simulink model "mav_project"  (R2024b)
settings: Solver=ode4  StartTime=0.0  StopTime=10000  RelTol=1e-3  EnableMultiTasking=on
model workspace (MAT data in the model file):
  P.gravity = 9.8
  P.mass = 1.56
  P.Jx = 0.1147
  P.Jy = 0.0576
  P.Jz = 0.1712
  P.Jxz = 0.0015
  P.M = 50
  P.epsilon = 0.1592
  P.alpha0 = 0.4712
  P.rho = 1.2682
  P.c = 0.3302
  P.b = 1.4224
  P.S_wing = 0.2589
  P.S_prop = 0.0314
  P.k_motor = 20
  P.C_L_0 = 0.28
  P.C_L_alpha = 3.45
  P.C_L_q = 0
  P.C_L_delta_e = -0.36
  P.C_D_0 = 0.03
  P.C_D_q = 0
  P.C_D_delta_e = 0
  P.C_M_0 = 0
  P.C_M_alpha = -0.38
  P.C_M_q = -3.6
  P.C_M_delta_e = -0.5
  P.C_Y_0 = 0
  P.C_Y_beta = -0.98
  P.C_Y_p = -0.26
  P.C_Y_r = 0
  P.C_Y_delta_a = 0
  P.C_Y_delta_r = -0.17
  P.C_ell_0 = 0
  P.C_ell_beta = -0.12
  P.C_ell_p = -0.26
  P.C_ell_r = 0.14
  P.C_ell_delta_a = 0.08
  P.C_ell_delta_r = 0.105
  P.C_n_0 = 0
  P.C_n_beta = 0.25
  P.C_n_p = 0.022
  P.C_n_r = -0.35
  P.C_n_delta_a = 0.06
  P.C_n_delta_r = -0.032
  P.C_prop = 1
  P.wind_n = 0
  P.wind_e = 0
  P.wind_d = 0
  P.L_wx = 1250
  P.L_wy = 1750
  P.L_wz = 1750
  P.sigma_wx = 1
  P.sigma_wy = 1
  P.sigma_wz = 1
  P.Va0 = 10
  P.Ts = 0.01
  P.Va = 13
  P.pn0 = 0
  P.pe0 = 0
  P.pd0 = 0
  P.u0 = 12.9669102518
  P.v0 = 3.28039918827e-26
  P.w0 = 0.926951196428
  P.phi0 = 1.93188396575e-23
  P.theta0 = 0.0713644980387
  P.psi0 = 4.37095971631e-18
  P.p0 = -4.12839964336e-24
  P.q0 = -1.29183976294e-24
  P.r0 = 9.37982436998e-24
  P.u_trim = [-0.0542370185094; 4.00408429765e-25; -1.10117211384e-23; 0.825366374251]
  P.x_trim = [5.38381030697e-18; -2.86631315328e-18; 3.31364444525e-19; 12.9669102518; 3.28039918827e-26; 0.926951196428; 1.93188396575e-23; 0.0713644980387; 4.37095971631e-18; -4.12839964336e-24; -1.29183976294e-24; 9.37982436998e-24]
  P.tau = 5
  P.altitude_take_off_zone = 10
  P.altitude_hold_zone = 10
  P.roll_kp = 2.56718517289
  P.roll_kd = 0.253887920845
  P.roll_ki = 0.1
  P.heading_kp = 1.58199403044
  P.heading_ki = 0.943612282481
  P.heading_kd = 0
  P.beta_kp = 0.116355283466
  P.beta_ki = 0
  P.beta_kd = 0
  P.pitch_kp = -1.36164063875
  P.pitch_kd = -0.139518937604
  P.pitch_ki = 0
  P.K_theta_DC = 0.641786650331
  P.altitude_kp = 0.0733804862104
  P.altitude_ki = 0.0224696538774
  P.altitude_kd = 0
  P.airspeed_pitch_kp = -0.208266228183
  P.airspeed_pitch_ki = -0.268260153434
  P.airspeed_pitch_kd = 0
  P.airspeed_throttle_kp = 12.4207118815
  P.airspeed_throttle_ki = 2.96647332332
  P.airspeed_throttle_kd = 0
  P.sideslip_kp = 0.1
  P.sideslip_kd = -0.5
  P.sideslip_ki = 0
values from neighbouring files (symbols this model uses):
  P = varargin{5}    [my_mav_dynamics.m]
undefined symbols (not defined in the file or in its folder): autopilot, drawAircraft, ekf_nav, forces_moments, gps_sensor, Guidance, imu_sensor, LQR_Controller, plotmavstatevariables, Receive, Send
libraries: simulink x6, aerolibanim x2, aerolibfltsims x2, slrealtimeiplib x1, vrlib x1
settings Model: SimulationMode=accelerator  Creator=beard  LastModifiedBy=solot
settings SolverCC: AutoInsertRateTranBlk=on
settings DataIOCC: LimitDataPoints=on  SaveFormat=Array  SignalLoggingSaveFormat=ModelDataLogs  ReturnWorkspaceOutputs=off
settings OptimizationCC: ExpressionDepthLimit=2147483647  InitFltsAndDblsToZero=on  LifeSpan=inf
settings DebuggingCC: SolverPrmCheckMsg=warning  FcnCallInpInsideContextMsg=warning  UnconnectedInputMsg=warning  UnconnectedOutputMsg=warning  UnconnectedLineMsg=warning  StateNameClashWarn=warning  SFUnexpectedBacktrackingDiag=warning  SFNoUnconditionalDefaultTransitionDiag=warning  SFExecutionAtInitializationDiag=none  ArithmeticOperatorsInVariantConditions=warning
settings HardwareCC: ProdBitPerPointer=32  ProdBitPerSizeT=32  ProdBitPerPtrDiffT=32  ProdLargestAtomicFloat=None  ProdIntDivRoundTo=Undefined  ProdEndianess=Unspecified  ProdWordSize=32  ProdHWDeviceType=32-bit Generic
settings ModelReferenceCC: EnableRefExpFcnMdlSchedulingChecks=on  PropagateSignalLabelsOutOfModel=off
settings SFSimCC: SimUseLocalCustomCode=off  CustomCodeUndefinedFunction=UseInterfaceOnly
settings RTWCC: RTWUseLocalCustomCode=off  GPUComputeCapability=3.5  DLArmComputeVersion=19.05
settings CodeAppCC: StateflowObjectComments=on
settings GRTTargetCC: TargetLangStandard=C89/C90 (ANSI)  CombineOutputUpdateFcns=off  GRTInterface=on
settings ConfigComp: CovMetricSettings=dw  CovSaveCumulativeToWorkspaceVar=on  CovSaveSingleToWorkspaceVar=on  CovExternalEMLEnable=off

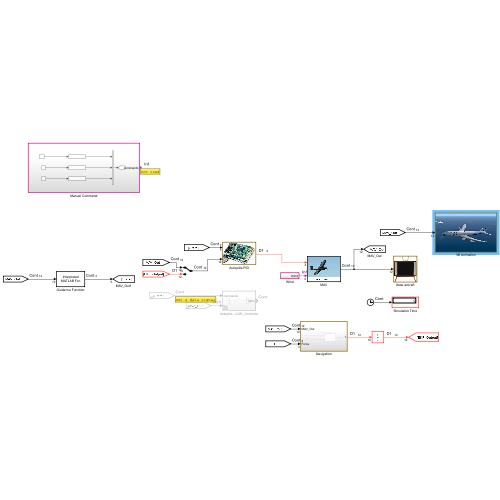
[thumbnail: Simulink's stored preview of the top-level diagram]
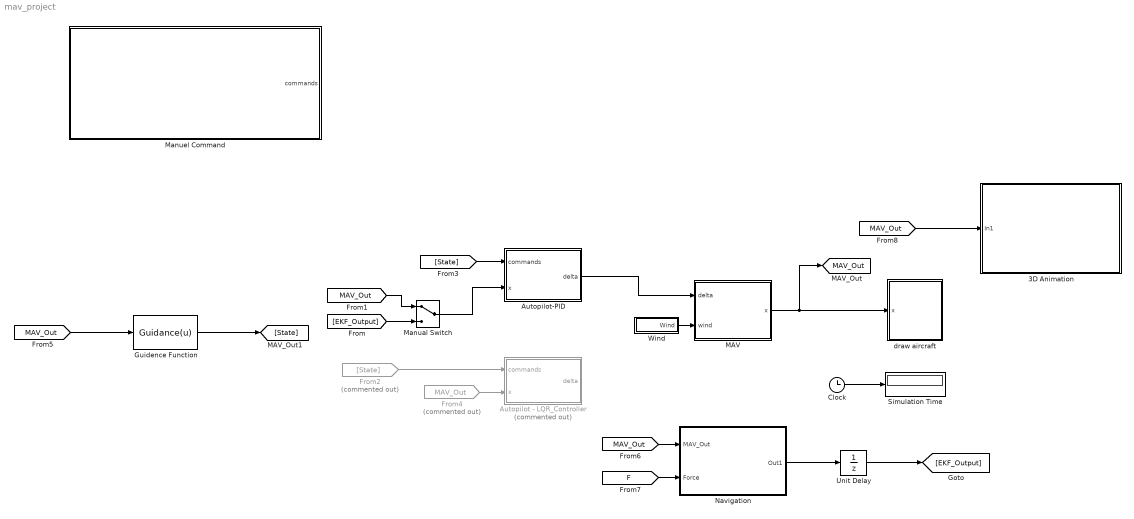
== system mav_project ==
  3D Animation : Subsystem
      mask Display: image(imread('flight.jpg'))
  Autopilot - LQR_Controller : Subsystem  Commented=on
  Autopilot-PID : Subsystem
      mask Display: image('kestrel.jpg')
  Clock : Clock
  From2 : From  Commented=on  GotoTag=State
  From4 : From  Commented=on  GotoTag=MAV_Out  TagVisibility=global
  Guidence Function : MATLABFcn  MATLABFcn=Guidance(u)  OutputDimensions=3
  MAV : Subsystem
      mask Display: image('batcam.png')
  Manual Switch : ManualSwitch
  "Manuel Command " : Subsystem
  Navigation : Subsystem
  Simulation Time : Display
  Unit Delay : UnitDelay  SampleTime=0.01  HasFrameUpgradeWarning=on
  Wind : Subsystem
  draw aircraft : Subsystem
      mask init:
      | % parameters for drawing aircraft
      |   % scale size
      |   size = 20;
      |   fuse_l1    = 7;
      |   fuse_l2    = 4;
      |   fuse_l3    = 15;
      |   fuse_w     = 2;
      |   wing_l     = 6;
      |   wing_w     = 20;
      |   tail_l     = 3;
      |   tail_h     = 3;
      |   tailwing_w = 10;
      |   tailwing_l = 3;
      |   % colors
      |   red     = [1, 0, 0];
      |   green   = [0, 1, 0];
      |   blue    = [0, 0, 1];
      |   yellow  = [1,1,0];
      |   magenta = [0, 1, 1];
      |   
      | 
      | % define vertices and faces for aircraft
      |   V = [...
      |     fuse_l1,             0,             0;...        % point 1
      |     fuse_l2,            -fuse_w/2,     -fuse_w/2;... % point 2     
      |     fuse_l2,             fuse_w/2,     -fuse_w/2;... % point 3     
      |     fuse_l2,             fuse_w/2,      fuse_w/2;... % point 4
      |     fuse_l2,            -fuse_w/2,      fuse_w/2;... % point 5
      |    -fuse_l3,             0,             0;...        % point 6
      |     0,                   wing_w/2,      0;...        % point 7
      |    -wing_l,              wing_w/2,      0;...        % point 8
      |    -wing_l,             -wing_w/2,      0;...        % point 9
      |     0,                  -wing_w/2,      0;...        % point 10
      |    -fuse_l3+tailwing_l,  tailwing_w/2,  0;...        % point 11
      |    -fuse_l3,             tailwing_w/2,  0;...        % point 12
      |    -fuse_l3,            -tailwing_w/2,  0;...        % point 13
      |    -fuse_l3+tailwing_l, -tailwing_w/2,  0;...        % point 14
      |    -fuse_l3+tailwing_l,  0,             0;...        % point 15
      |    -fuse_l3+tailwing_l,  0,             -tail_h;...  % point 16
      |    -fuse_l3,             0,             -tail_h;...  % point 17
      |   ];
      |   
      |   F = [...
      |         1,  2,  3,  1;... % nose-top
      |         1,  3,  4,  1;... % nose-left
      |         1,  4,  5,  1;... % nose-bottom
      |         1,  5,  2,  1;... % nose-right
      |         2,  3,  6,  2;... % fuselage-top
      |         3,  6,  4,  3;... % fuselage-left
      |         4,  6,  5,  4;... % fuselage-bottom
      |         2,  5,  6,  2;... % fuselage-right
      |         7,  8,  9, 10;... % wing
      |        11, 12, 13, 14;... % tailwing
      |         6, 15, 17, 17;... % tail
      |         
      |   ];  
      |   
      |   colors = [...
      |         yellow;... % nose-top
      |         yellow;... % nose-left
      |         yellow;... % nose-bottom
      |         yellow;... % nose-right
      |         blue;... % fuselage-top
      |         blue;... % fuselage-left
      |         red;... % fuselage-bottom
      |         blue;... % fuselage-right
      |         green;... % wing
      |         green;... % tailwing
      |         blue;... % tail
      |     ];
      | 
      |   V = size*V;   % rescale vertices
      mask Display: image('tv.jpg')
  tag scope: MAV_Out=global
  wires:
  Clock/1 -> Simulation Time/1
  Wind/1(Wind) -> MAV/2(wind)
  MAV/1(x) -> [MAV_Out], draw aircraft/1(x)
  [MAV_Out] -> Guidence Function/1
  From4/1 -> Autopilot - LQR_Controller/2(x)
  Guidence Function/1 -> [State]
  [MAV_Out] -> Navigation/1(MAV_Out)
  [F] -> Navigation/2(Force)
  Navigation/1(Out1) -> Unit Delay/1
  Unit Delay/1 -> [EKF_Output]
  [State] -> Autopilot-PID/1(commands)
  Manual Switch/1 -> Autopilot-PID/2(x)
  [EKF_Output] -> Manual Switch/2
  [MAV_Out] -> Manual Switch/1
  From2/1 -> Autopilot - LQR_Controller/1(commands)
  Autopilot-PID/1(delta) -> MAV/1(delta)
  [MAV_Out] -> 3D Animation/1(In1)

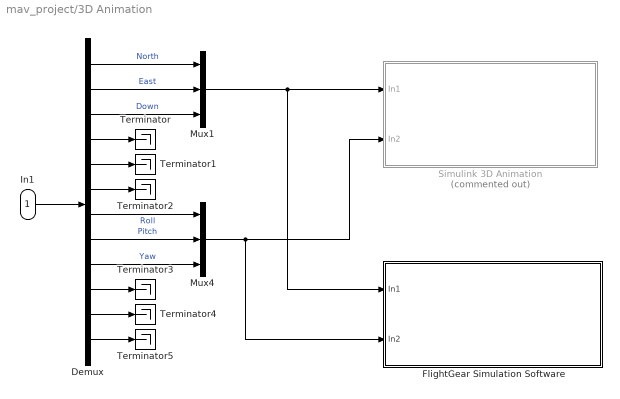
== system mav_project/3D Animation ==
  In1 : Inport
  Demux : Demux  Outputs=12
  FlightGear Simulation Software : Subsystem
      mask Display: image(imread('flightgear.jpg'))
  Mux1 : Mux  Inputs=3
  Mux4 : Mux  Inputs=3
  Simulink 3D Animation : Subsystem  Commented=on
      mask Display: image(imread('3danimation.JPG'))
  Terminator{,1..5} (6 alike) : Terminator
  wires:
  In1/1 -> Demux/1
  Demux/4 -> Terminator/1
  Demux/5 -> Terminator1/1
  Demux/6 -> Terminator2/1
  Demux/10 -> Terminator3/1
  Demux/11 -> Terminator4/1
  Demux/12 -> Terminator5/1
  Demux/1 -> Mux1/1  "North"
  Demux/2 -> Mux1/2  "East"
  Demux/3 -> Mux1/3  "Down"
  Mux1/1 -> FlightGear Simulation Software/1(In1), Simulink 3D Animation/1(In1)
  Demux/7 -> Mux4/1  "Roll"
  Demux/8 -> Mux4/2  "Pitch"
  Demux/9 -> Mux4/3  "Yaw"
  Mux4/1 -> FlightGear Simulation Software/2(In2), Simulink 3D Animation/2(In2)

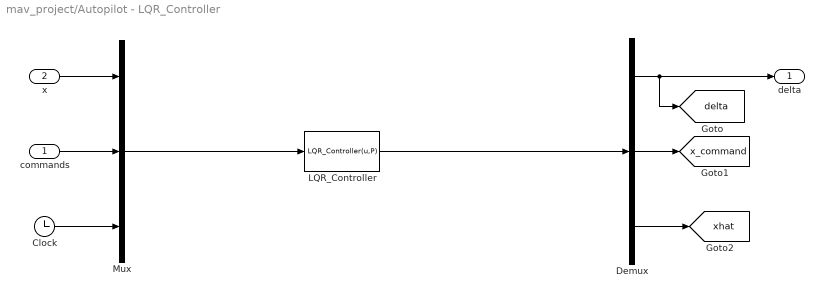
== system mav_project/Autopilot - LQR_Controller ==
  commands : Inport
  x : Inport  Port=2
  Clock : Clock
  Demux : Demux  Outputs=[4;12;12]
  LQR_Controller : MATLABFcn  MATLABFcn=LQR_Controller(u,P)  OutputDimensions=4+12+12
  Mux : Mux  Inputs=3
  delta : Outport
  tag scope: delta=global, x_command=global, xhat=global
  wires:
  Mux/1 -> LQR_Controller/1
  Demux/1 -> delta/1, [delta]
  Demux/3 -> [xhat]
  Demux/2 -> [x_command]
  Clock/1 -> Mux/3
  LQR_Controller/1 -> Demux/1
  commands/1 -> Mux/2
  x/1 -> Mux/1

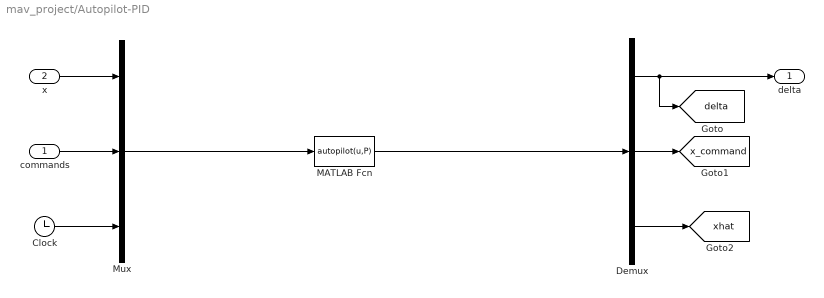
== system mav_project/Autopilot-PID ==
  commands : Inport
  x : Inport  Port=2
  Clock : Clock
  Demux : Demux  Outputs=[4;12;12]
  MATLAB Fcn : MATLABFcn  MATLABFcn=autopilot(u,P)  OutputDimensions=4+12+12  SampleTime=P.Ts
  Mux : Mux  Inputs=3
  delta : Outport
  tag scope: delta=global, x_command=global, xhat=global
  wires:
  Mux/1 -> MATLAB Fcn/1
  Clock/1 -> Mux/3
  MATLAB Fcn/1 -> Demux/1
  Demux/1 -> delta/1, [delta]
  Demux/2 -> [x_command]
  Demux/3 -> [xhat]
  x/1 -> Mux/1
  commands/1 -> Mux/2

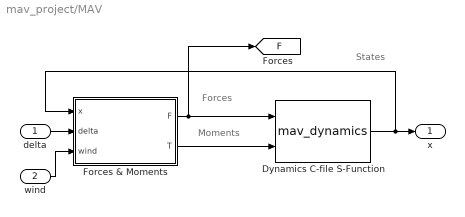
== system mav_project/MAV ==
  note: Forces
  note: Moments
  note: States
  delta : Inport
  wind : Inport  Port=2
  Dynamics C-file S-Function : S-Function  FunctionName=mav_dynamics  Parameters=mass,Jx,Jy,Jz,Jxz,pn0,pe0,pd0,u0,v0,w0,phi0,theta0,psi0,p0,q0,r0  SFunctionDeploymentMode=off  EnableBusSupport=off  mask{mass=P.mass, Jx=P.Jx, Jy=P.Jy, Jz=P.Jz, Jxz=P.Jxz, pn0=P.pn0, pe0=P.pe0, pd0=P.pd0, u0=P.u0, v0=P.v0, w0=P.w0, phi0=P.phi0, theta0=P.theta0, psi0=P.psi0, p0=P.p0, q0=P.q0, r0=P.r0}
      mask prompts: pn0 "Initial North position"; pe0 "Initial East position"; pd0 "Initial Down position"; u0 "Initial velocy u0"; v0 "Initial velocity v0"; w0 "Initial velocity w0"; phi0 "Initial roll angle"; theta0 "Initial pitch angle"; psi0 "Initial yaw angle"; p0 "Initial roll rate"; q0 "Initial pitch rate"; r0 "Initial yaw rate"
  Forces & Moments : Subsystem
  x : Outport
  tag scope: F=global
  wires:
  Dynamics C-file S-Function/1 -> Forces & Moments/1(x), x/1
  Forces & Moments/1(F) -> [F], Dynamics C-file S-Function/1
  Forces & Moments/2(T) -> Dynamics C-file S-Function/2
  delta/1 -> Forces & Moments/2(delta)
  wind/1 -> Forces & Moments/3(wind)

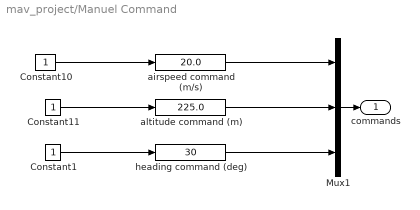
== system mav_project/Manuel Command  ==
  Constant1 : Constant
  Constant10 : Constant
  Constant11 : Constant
  Mux1 : Mux  Inputs=3
  airspeed command (m/s) : simulink/Math Operations/Slider Gain  gain=20.0  low=0  high=20
  altitude command (m) : simulink/Math Operations/Slider Gain  gain=225.0  low=0  high=500
  heading command (deg) : simulink/Math Operations/Slider Gain  gain=30  low=-360  high=360
  commands : Outport
  wires:
  Constant11/1 -> altitude command (m)/1
  heading command (deg)/1 -> Mux1/3
  Constant10/1 -> airspeed command (m/s)/1
  Mux1/1 -> commands/1
  altitude command (m)/1 -> Mux1/2
  airspeed command (m/s)/1 -> Mux1/1
  Constant1/1 -> heading command (deg)/1

== system mav_project/Navigation ==
  MAV_Out : Inport
  Force : Inport  Port=2
  Pulse Generator : DiscretePulseGenerator  PulseType=Time based  Period=1  PulseWidth=50
  Triggered Subsystem : Subsystem  TreatAsAtomicUnit=on
  Out1 : Outport
  wires:
  Pulse Generator/1 -> Triggered Subsystem/Trigger
  MAV_Out/1 -> Triggered Subsystem/1(MAV_Out)
  Force/1 -> Triggered Subsystem/2(Force)
  Triggered Subsystem/1(Out1) -> Out1/1

== system mav_project/Wind ==
  Constant1 : Constant  Value=[0; 0; 0]
  Constant2 : Constant  Value=[P.wind_n; P.wind_e; P.wind_d]
  Mux1 : Mux  Inputs=2
  Wind Gusts : Subsystem  Commented=on
  Wind : Outport
  wires:
  Constant2/1 -> Mux1/1
  Mux1/1 -> Wind/1
  Constant1/1 -> Mux1/2

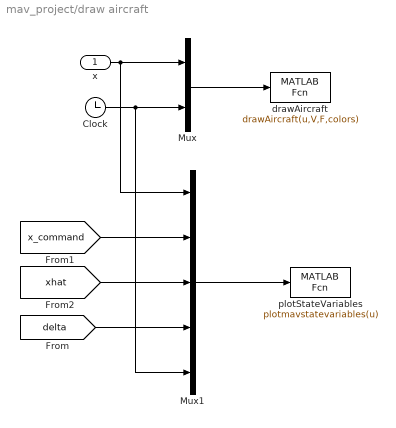
== system mav_project/draw aircraft ==
  x : Inport
  Clock : Clock
  Mux : Mux  Inputs=2
  Mux1 : Mux  Inputs=5
  drawAircraft : MATLABFcn  MATLABFcn=drawAircraft(u,V,F,colors)  OutputDimensions=0  SampleTime=0.1
  plotStateVariables : MATLABFcn  MATLABFcn=plotmavstatevariables(u)  OutputDimensions=0  SampleTime=0.1
  wires:
  Mux/1 -> drawAircraft/1
  x/1 -> Mux/1, Mux1/1
  Clock/1 -> Mux/2, Mux1/5
  Mux1/1 -> plotStateVariables/1
  [xhat] -> Mux1/3
  [x_command] -> Mux1/2
  [delta] -> Mux1/4

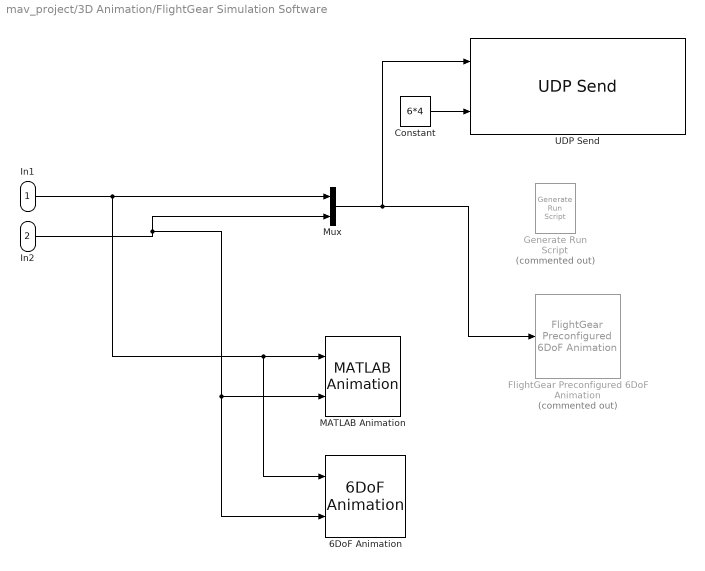
== system mav_project/3D Animation/FlightGear Simulation Software ==
  In1 : Inport
  In2 : Inport  Port=2
  6DoF Animation : aerolibanim/6DoF Animation  u1=[0 4000 -2000 2000 -5000 -3000]  u2=0.1  u3=1.0  u4=[4000 0 -5000]  u5=Fixed position  u6=[2000 500 -3150]  u7=10  u8=on
  Constant : Constant  Value=6*4
  FlightGear Preconfigured 6DoF Animation : aerolibfltsims/FlightGear Preconfigured 6DoF Animation  Commented=on  xFlightGearVersion=v2016.1  DestinationIpAddress=127.0.0.1  DestinationPort=5502  SampleTime=1/100  packetVersion=24
  Generate Run Script : aerolibfltsims/Generate Run Script  Commented=on  Architecture=Default  dataFlow=Send-Receive  GeometryModelName=c172p  AirportId=KSFO  RunwayId=10L  InitialAltitude=7224  InitialHeading=113  OffsetDistance=4.72  OffsetAzimuth=0  InstallScenery=off  DisableShaders=off  OriginAddress=127.0.0.1  DestinationPort=5502  OriginPort=5505  LocalAddress=127.0.0.1  OutputFileName=runfg.bat  FlightGearBaseDirectory=C:\Program Files\FlightGear 2024.1
  MATLAB Animation : aerolibanim/MATLAB Animation  Tag=Matlab Animation 6 DOF  Vehicles=1  Geometries='astredwedge.mat'  BoundingBoxCoordinates=[-50,50,-50,50,-50,50]  CameraOffset=[-150,-50,0]  CameraViewAngle=3  SampleTime=0.2  FigurePosition=[5.482000e+02,1.778000e+02,3.816000e+02,3.352000e+02]
  Mux : Mux  Inputs=2
  UDP Send : slrealtimeiplib/UDP Send  useHostTargetConn=off  toAddress='127.0.0.1'  toPort=5502  sampleTime=0.01  enableMessage=off
  wires:
  In2/1 -> 6DoF Animation/2, MATLAB Animation/2, Mux/2
  In1/1 -> Mux/1, 6DoF Animation/1, MATLAB Animation/1
  Mux/1 -> UDP Send/1, FlightGear Preconfigured 6DoF Animation/1
  Constant/1 -> UDP Send/2

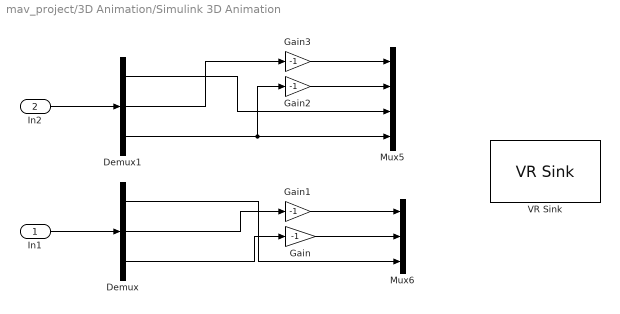
== system mav_project/3D Animation/Simulink 3D Animation ==
  In1 : Inport
  In2 : Inport  Port=2
  Demux : Demux  Outputs=3
  Demux1 : Demux  Outputs=3
  Gain{,1..3} (4 alike) : Gain  Gain=-1
  Mux5 : Mux
  Mux6 : Mux  Inputs=3
  VR Sink : vrlib/VR Sink  InstantiateOnLoad=on  SampleTime=0.05  ViewEnable=on  RemoteChange=off  RemoteView=off  WorldFileName=b748.wrl  WorldDescription=B747 Flying over the San Francisco Area  AutoView=on  VideoDimensions=[]  AllowVariableSize=off
  wires:
  Gain3/1 -> Mux5/1
  Gain1/1 -> Mux6/1
  Gain2/1 -> Mux5/2
  Gain/1 -> Mux6/2
  Demux/3 -> Gain/1
  Demux1/3 -> Gain2/1, Mux5/4
  Demux1/2 -> Gain3/1
  Demux1/1 -> Mux5/3
  Demux/1 -> Mux6/3
  Demux/2 -> Gain1/1
  In1/1 -> Demux/1
  In2/1 -> Demux1/1

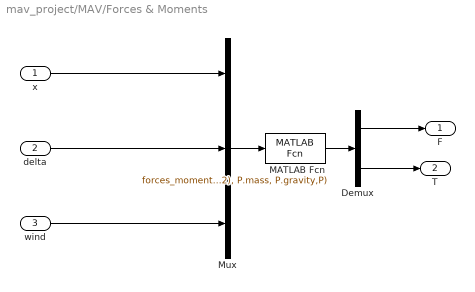
== system mav_project/MAV/Forces & Moments ==
  x : Inport
  delta : Inport  Port=2
  wind : Inport  Port=3
  Demux : Demux  Outputs=2
  MATLAB Fcn : MATLABFcn  MATLABFcn=forces_moments(u(1:12),u(13:16),u(17:22), P.mass, P.gravity,P)  OutputDimensions=6
  Mux : Mux  Inputs=3
  F : Outport
  T : Outport  Port=2
  wires:
  x/1 -> Mux/1
  delta/1 -> Mux/2
  wind/1 -> Mux/3
  MATLAB Fcn/1 -> Demux/1
  Demux/1 -> F/1
  Demux/2 -> T/1
  Mux/1 -> MATLAB Fcn/1

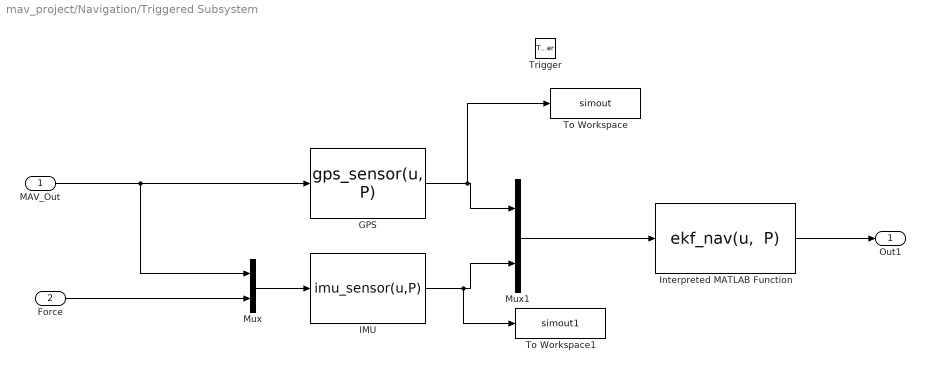
== system mav_project/Navigation/Triggered Subsystem ==
  MAV_Out : Inport
  Force : Inport  Port=2
  Trigger : TriggerPort  VariantControl=(inherit)
  GPS : MATLABFcn  MATLABFcn=gps_sensor(u, P)  OutputDimensions=5
  IMU : MATLABFcn  MATLABFcn=imu_sensor(u,P)  OutputDimensions=6
  Interpreted MATLAB Function : MATLABFcn  MATLABFcn="ekf_nav(u,  P)"  OutputDimensions=12
  Mux : Mux  Inputs=2
  Mux1 : Mux  Inputs=2
  To Workspace : ToWorkspace  VariableName=simout  SaveFormat=Structure  SampleTime=-1
  To Workspace1 : ToWorkspace  VariableName=simout1  SaveFormat=Structure  SampleTime=-1
  Out1 : Outport
  wires:
  GPS/1 -> To Workspace/1, Mux1/1
  Interpreted MATLAB Function/1 -> Out1/1
  IMU/1 -> To Workspace1/1, Mux1/2
  Mux/1 -> IMU/1
  Mux1/1 -> Interpreted MATLAB Function/1
  MAV_Out/1 -> Mux/1, GPS/1
  Force/1 -> Mux/2

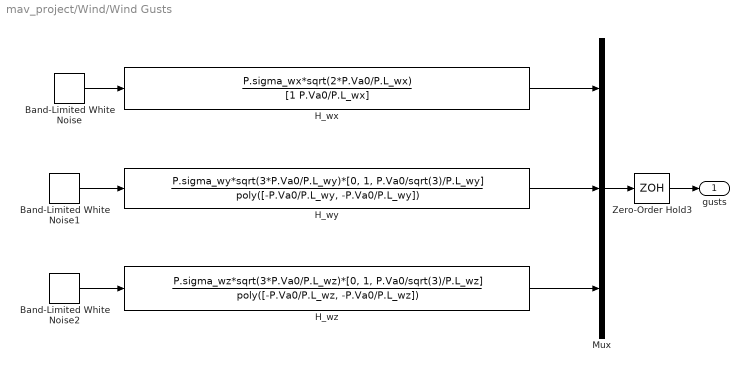
== system mav_project/Wind/Wind Gusts ==
  Band-Limited White Noise : simulink/Sources/Band-Limited White Noise  Cov=[1]  Ts=P.Ts  seed=[23341]
  Band-Limited White Noise1 : simulink/Sources/Band-Limited White Noise  Cov=[1]  Ts=P.Ts  seed=[23341]
  Band-Limited White Noise2 : simulink/Sources/Band-Limited White Noise  Cov=[1]  Ts=P.Ts  seed=[23341]
  H_wx : TransferFcn  Numerator=P.sigma_wx*sqrt(2*P.Va0/P.L_wx)  Denominator=[1 P.Va0/P.L_wx]
  H_wy : TransferFcn  Numerator=P.sigma_wy*sqrt(3*P.Va0/P.L_wy)*[0, 1, P.Va0/sqrt(3)/P.L_wy]  Denominator=poly([-P.Va0/P.L_wy, -P.Va0/P.L_wy])
  H_wz : TransferFcn  Numerator=P.sigma_wz*sqrt(3*P.Va0/P.L_wz)*[0, 1, P.Va0/sqrt(3)/P.L_wz]  Denominator=poly([-P.Va0/P.L_wz, -P.Va0/P.L_wz])
  Mux : Mux  Inputs=3
  Zero-Order Hold3 : ZeroOrderHold  SampleTime=P.Ts
  gusts : Outport
  wires:
  H_wx/1 -> Mux/1
  Band-Limited White Noise/1 -> H_wx/1
  H_wy/1 -> Mux/2
  Band-Limited White Noise1/1 -> H_wy/1
  H_wz/1 -> Mux/3
  Band-Limited White Noise2/1 -> H_wz/1
  Mux/1 -> Zero-Order Hold3/1
  Zero-Order Hold3/1 -> gusts/1
